simulink model "uklad03"  (R2024a)
settings: Solver=VariableStepAuto  StartTime=0.0  StopTime=10  RelTol=1e-3
settings Model: Creator=kwisniew  LastModifiedBy=kwisniew
settings DataIOCC: ReturnWorkspaceOutputs=off

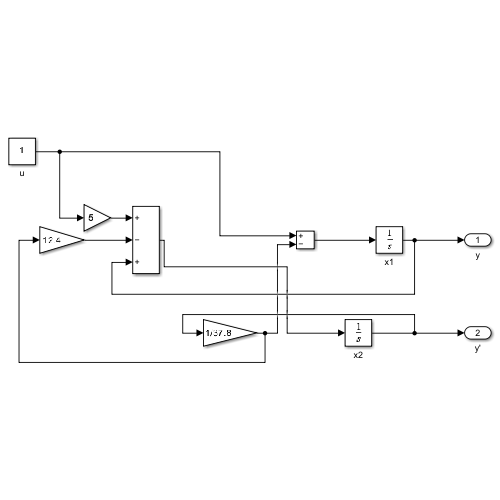
[thumbnail: Simulink's stored preview of the top-level diagram]
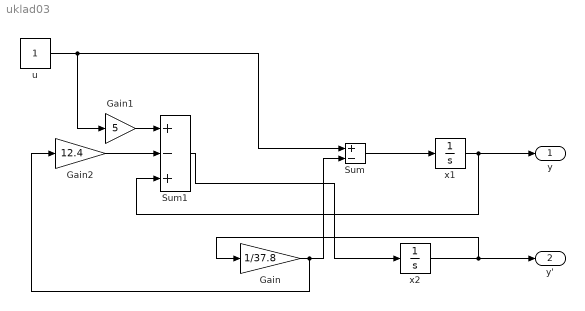
== system uklad03 ==
  Gain : Gain  Gain=1/37.8
  Gain1 : Gain  Gain=5
  Gain2 : Gain  Gain=12.4
  Sum : Sum  Inputs=+-
  Sum1 : Sum  Inputs=+-+
  u : Constant
  x1 : Integrator  InitialCondition=0.5
  x2 : Integrator  InitialCondition=0.1
  y : Outport
  y' : Outport  Port=2
  wires:
  x2/1 -> Gain/1, y'/1
  x1/1 -> Sum1/3, y/1
  Gain/1 -> Gain2/1, Sum/2
  u/1 -> Gain1/1, Sum/1
  Sum/1 -> x1/1
  Gain1/1 -> Sum1/1
  Gain2/1 -> Sum1/2
  Sum1/1 -> x2/1
